simulink model "NREL5MW_Baseline_loads_IPC_1P_v3_2014b"  (R2014b)
settings: Solver=ode3  SolverMode=SingleTasking  StartTime=0.0  StopTime=T-76  RelTol=1e-3
InitFcn:
  | Simsetup
undefined symbols (not defined in the file or in its folder): delta_1p, Demanded_torque, dLP, dLPP, DT, Gainn, IPC_Pitch_max, k_1p, ki_1p, Kp, Mode_gain, NDOF, NumOuts, omega_1p, omega_B, omega_C, omega_L, OutList, PA, Pitch_fine, Pitch_max, Pitch_max_rate, Pitch_min, Pitch_min_rate, PKp, PTi, q_init, qdot_init, strmatch, Ti, Torque_limit, Torque_slew_rate, zeta_1p, zeta_L
libraries: simulink x5
settings Model: ExtModeTrigMode=oneshot  ExtModeArmWhenConnect=off  Creator=Hazim Namik  LastModifiedBy=bwilson
settings OptimizationCC: BlockReduction=off  BooleanDataType=off
settings DebuggingCC: SaveWithParameterizedLinksMsg=none  UnderspecifiedInitializationDetection=Classic  MergeDetectMultiDrivingBlocksExec=none  SignalResolutionControl=TryResolveAllWithWarning  SolverPrmCheckMsg=none  FrameProcessingCompatibilityMsg=error
settings HardwareCC: TargetUnknown=on

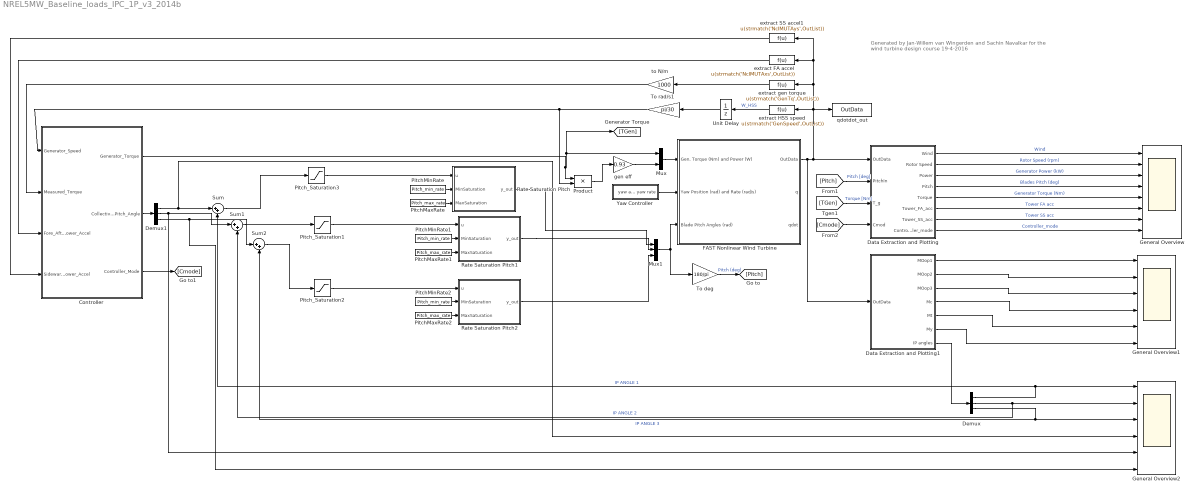
== system NREL5MW_Baseline_loads_IPC_1P_v3_2014b ==
  note: Generated by Jan-Willem van Wingerden and Sachin Navalkar
      | for the wind turbine design course 19-4-2016
  Controller : Subsystem
  Data Extraction and Plotting : Subsystem
  Data Extraction and Plotting1 : Subsystem
  Demux : Demux  Outputs=3
  Demux1 : Demux  Outputs=3
  FAST Nonlinear Wind Turbine : Subsystem  mask(FAST Nonlinear Wind Turbine){}
      mask help: This block contains the FAST S-Function and blocks that integrate the DOF accelerations to get velocities and displacements.
      mask init:
      | clear FAST_SFunc
      settings: MinAlgLoopOccurrences=on
  General Overview : Scope  NumInputPorts=8
      settings: TickLabels=on  YMin=4.47125~10.53034~-754.23394~-1.76549~-5387.5~-3.12398~-0.52601~1.625  YMax=24.47125~15.22691~6788.10547~16.63959~48487.5~2.86069~0.51885~5.375  SaveName=ScopeData2
  General Overview1 : Scope  NumInputPorts=6
      settings: TickLabels=on  YMin=-3775.82161~-2417.73125~-6271.52916~-2978.12919~-4139.15524~-3775.35224  YMax=17382.79924~16229.60392~17181.20499~16116.4566~2206.392~3982.30783
  General Overview2 : Scope  NumInputPorts=6
      settings: TickLabels=on  YMin=-0.04911~-0.0435~-0.0444~-0.02537~-0.02537~-0.02537  YMax=0.04183~0.04676~0.0485~0.24679~0.24679~0.24679
  Mux : Mux  Inputs=2
  Mux1 : Mux  Inputs=3
  PitchMaxRate : Constant  Value=Pitch_max_rate
  PitchMaxRate1 : Constant  Value=Pitch_max_rate
  PitchMaxRate2 : Constant  Value=Pitch_max_rate
  PitchMinRate : Constant  Value=Pitch_min_rate
  PitchMinRate1 : Constant  Value=Pitch_min_rate
  PitchMinRate2 : Constant  Value=Pitch_min_rate
  Pitch_Saturation1 : Saturate  UpperLimit=Pitch_max*pi/180  LowerLimit=Pitch_min*pi/180
  Pitch_Saturation2 : Saturate  UpperLimit=Pitch_max*pi/180  LowerLimit=Pitch_min*pi/180
  Pitch_Saturation3 : Saturate  UpperLimit=Pitch_max*pi/180  LowerLimit=Pitch_min*pi/180
  Product : Product  RndMeth=Zero
  Rate Saturation Pitch : MATLAB Function  TreatAsAtomicUnit=on
  Rate Saturation Pitch1 : MATLAB Function  TreatAsAtomicUnit=on
  Rate Saturation Pitch2 : MATLAB Function  TreatAsAtomicUnit=on
  Sum : Sum  Inputs=|++
  Sum1 : Sum  Inputs=|++
  Sum2 : Sum  Inputs=|++
  To deg : Gain  Gain=180/pi
  To rad/s1 : Gain  Gain=pi/30
  Unit Delay : UnitDelay  InitialCondition=12.1*97  SampleTime=0.0125
  Yaw Controller : Subsystem
  extract FA accel : Fcn  Expr=u(strmatch('NcIMUTAxs',OutList))
  extract HSS speed : Fcn  Expr=u(strmatch('GenSpeed',OutList))
  extract SS accel1 : Fcn  Expr=u(strmatch('NcIMUTAys',OutList))
  extract gen torque : Fcn  Expr=u(strmatch('GenTq',OutList))
  gen eff : Gain  Gain=0.93
  qdotdot_out : ToWorkspace  VariableName=OutData  SampleTime=-1
  to N/m : Gain  Gain=1000
  wires:
  Mux/1 -> FAST Nonlinear Wind Turbine/1(Gen. Torque (Nm) and Power (W))
  Yaw Controller/1(yaw and yaw rate) -> FAST Nonlinear Wind Turbine/2(Yaw Position (rad) and Rate (rad/s))
  extract HSS speed/1 -> Unit Delay/1  "W_HSS"
  To deg/1 -> [Pitch]  "Pitch (deg)"
  gen eff/1 -> Mux/2
  Product/1 -> gen eff/1
  To rad/s1/1 -> Controller/1(Generator_Speed), Product/2
  Data Extraction and Plotting/3(Power) -> General Overview/3  "Generator Power (kW)"
  [Pitch] -> Data Extraction and Plotting/2(PitchIn)  "Pitch [deg]"
  Data Extraction and Plotting/1(Wind) -> General Overview/1  "Wind"
  Data Extraction and Plotting/2(Rotor Speed) -> General Overview/2  "Rotor Speed (rpm)"
  [TGen] -> Data Extraction and Plotting/3(T_g)  "Torque [Nm]"
  FAST Nonlinear Wind Turbine/1(OutData) -> Data Extraction and Plotting1/1(OutData), Data Extraction and Plotting/1(OutData), extract SS accel1/1, extract FA accel/1, extract gen torque/1, extract HSS speed/1, qdotdot_out/1
  Data Extraction and Plotting/4(Pitch) -> General Overview/4  "Blades Pitch (deg)"
  Data Extraction and Plotting/5(Torque) -> General Overview/5  "Generator Torque (Nm)"
  Unit Delay/1 -> To rad/s1/1
  extract gen torque/1 -> to N/m/1
  to N/m/1 -> Controller/2(Measured_Torque)
  Controller/1(Generator_Torque) -> Mux/1, [TGen], Product/1
  extract FA accel/1 -> Controller/3(Fore_Aft_Tower_Accel)
  extract SS accel1/1 -> Controller/4(Sidewards_Tower_Accel)
  Data Extraction and Plotting/6(Tower_FA_acc) -> General Overview/6  "Tower FA acc"
  Data Extraction and Plotting/7(Tower_SS_acc) -> General Overview/7  "Tower SS acc"
  Controller/3(Controller_Mode) -> [Cmode]
  [Cmode] -> Data Extraction and Plotting/4(Cmod)
  Data Extraction and Plotting/8(Controller_mode) -> General Overview/8  "Controller_mode"
  Data Extraction and Plotting1/1(MOop1) -> General Overview1/1
  Data Extraction and Plotting1/2(MOop2) -> General Overview1/2
  Data Extraction and Plotting1/3(MOop3) -> General Overview1/3
  Data Extraction and Plotting1/4(Mc) -> General Overview1/4
  Data Extraction and Plotting1/5(Mt) -> General Overview1/5
  Data Extraction and Plotting1/6(My) -> General Overview1/6
  Data Extraction and Plotting1/7(IP angles) -> Demux/1
  Demux/1 -> Sum/2, General Overview2/1  "IP ANGLE 1"
  Demux/2 -> Sum1/2, General Overview2/2  "IP ANGLE 2"
  Demux/3 -> General Overview2/3, Sum2/2  "IP ANGLE 3"
  Controller/2(Collective_Pitch_Angle) -> Demux1/1
  Demux1/1 -> General Overview2/4, Sum/1
  Demux1/2 -> General Overview2/5, Sum1/1
  Demux1/3 -> General Overview2/6, Sum2/1
  Mux1/1 -> To deg/1, FAST Nonlinear Wind Turbine/3(Blade Pitch Angles (rad))
  Rate Saturation Pitch/1(y_out) -> Mux1/1
  Sum1/1 -> Pitch_Saturation1/1
  Rate Saturation Pitch1/1(y_out) -> Mux1/2
  Rate Saturation Pitch2/1(y_out) -> Mux1/3
  Sum/1 -> Pitch_Saturation3/1
  PitchMinRate/1 -> Rate Saturation Pitch/2(MinSaturation)
  PitchMaxRate/1 -> Rate Saturation Pitch/3(MaxSaturation)
  Pitch_Saturation3/1 -> Rate Saturation Pitch/1(u)
  PitchMinRate1/1 -> Rate Saturation Pitch1/2(MinSaturation)
  PitchMaxRate1/1 -> Rate Saturation Pitch1/3(MaxSaturation)
  Pitch_Saturation1/1 -> Rate Saturation Pitch1/1(u)
  Sum2/1 -> Pitch_Saturation2/1
  PitchMinRate2/1 -> Rate Saturation Pitch2/2(MinSaturation)
  PitchMaxRate2/1 -> Rate Saturation Pitch2/3(MaxSaturation)
  Pitch_Saturation2/1 -> Rate Saturation Pitch2/1(u)

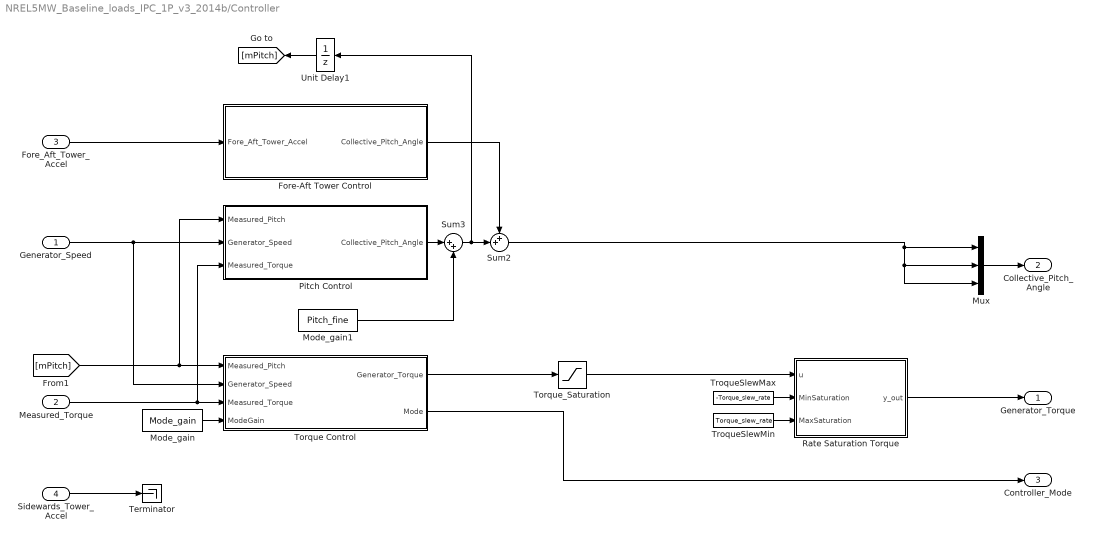
== system NREL5MW_Baseline_loads_IPC_1P_v3_2014b/Controller ==
  Generator_Speed : Inport
  Measured_Torque : Inport  Port=2
  Fore_Aft_Tower_Accel : Inport  Port=3
  Sidewards_Tower_Accel : Inport  Port=4  PortDimensions=1
  Fore-Aft Tower Control : Subsystem
  Mode_gain : Constant  Value=Mode_gain
  Mode_gain1 : Constant  Value=Pitch_fine
  Mux : Mux  Inputs=3
  Pitch Control : Subsystem
  Rate Saturation Torque : MATLAB Function  TreatAsAtomicUnit=on
  Sum2 : Sum  Inputs=++|
  Sum3 : Sum  Inputs=|++
  Terminator : Terminator
  Torque Control : Subsystem
  Torque_Saturation : Saturate  UpperLimit=Torque_limit  LowerLimit=0
  TroqueSlewMax : Constant  Value=-Torque_slew_rate
  TroqueSlewMin : Constant  Value=Torque_slew_rate
  Unit Delay1 : UnitDelay  InitialCondition=12.1*97  SampleTime=DT
  Generator_Torque : Outport
  Collective_Pitch_Angle : Outport  Port=2  PortDimensions=3
  Controller_Mode : Outport  Port=3  PortDimensions=1
  wires:
  Sidewards_Tower_Accel/1 -> Terminator/1
  Fore_Aft_Tower_Accel/1 -> Fore-Aft Tower Control/1(Fore_Aft_Tower_Accel)
  Fore-Aft Tower Control/1(Collective_Pitch_Angle) -> Sum2/1
  Rate Saturation Torque/1(y_out) -> Generator_Torque/1
  [mPitch] -> Pitch Control/1(Measured_Pitch), Torque Control/1(Measured_Pitch)
  Measured_Torque/1 -> Torque Control/3(Measured_Torque), Pitch Control/3(Measured_Torque)
  Generator_Speed/1 -> Pitch Control/2(Generator_Speed), Torque Control/2(Generator_Speed)
  Mode_gain/1 -> Torque Control/4(ModeGain)
  Torque Control/1(Generator_Torque) -> Torque_Saturation/1
  Mux/1 -> Collective_Pitch_Angle/1
  Unit Delay1/1 -> [mPitch]
  Torque Control/2(Mode) -> Controller_Mode/1
  Mode_gain1/1 -> Sum3/2
  Pitch Control/1(Collective_Pitch_Angle) -> Sum3/1
  Sum3/1 -> Sum2/2, Unit Delay1/1
  Sum2/1 -> Mux/2, Mux/3, Mux/1
  Torque_Saturation/1 -> Rate Saturation Torque/1(u)
  TroqueSlewMax/1 -> Rate Saturation Torque/2(MinSaturation)
  TroqueSlewMin/1 -> Rate Saturation Torque/3(MaxSaturation)

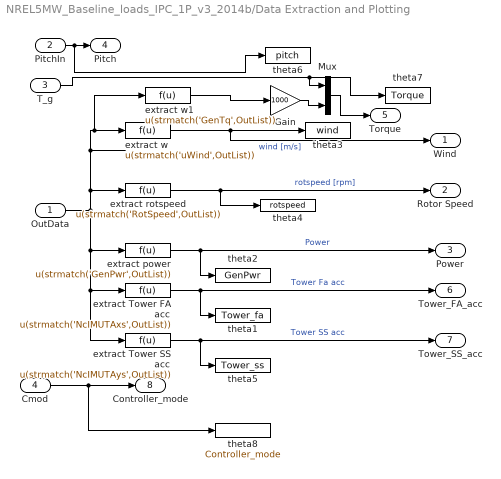
== system NREL5MW_Baseline_loads_IPC_1P_v3_2014b/Data Extraction and Plotting ==
  OutData : Inport
  PitchIn : Inport  Port=2
  T_g : Inport  Port=3
  Cmod : Inport  Port=4
  Gain : Gain  Gain=1000
  Mux : Mux  Inputs=2
  extract Tower FA acc : Fcn  Expr=u(strmatch('NcIMUTAxs',OutList))
  extract Tower SS acc : Fcn  Expr=u(strmatch('NcIMUTAys',OutList))
  extract power : Fcn  Expr=u(strmatch('GenPwr',OutList))
  extract rotspeed : Fcn  Expr=u(strmatch('RotSpeed',OutList))
  extract w : Fcn  Expr=u(strmatch('uWind',OutList))
  extract w1 : Fcn  Expr=u(strmatch('GenTq',OutList))
  theta1 : ToWorkspace  VariableName=Tower_fa
      settings: MaxDataPoints=Inf
  theta2 : ToWorkspace  VariableName=GenPwr
      settings: MaxDataPoints=Inf
  theta3 : ToWorkspace  VariableName=wind
      settings: MaxDataPoints=Inf
  theta4 : ToWorkspace  VariableName=rotspeed
      settings: MaxDataPoints=Inf
  theta5 : ToWorkspace  VariableName=Tower_ss
      settings: MaxDataPoints=Inf
  theta6 : ToWorkspace  VariableName=pitch
      settings: MaxDataPoints=Inf
  theta7 : ToWorkspace  VariableName=Torque
      settings: MaxDataPoints=Inf
  theta8 : ToWorkspace  VariableName=Controller_mode
      settings: MaxDataPoints=Inf
  Wind : Outport
  Rotor Speed : Outport  Port=2
  Power : Outport  Port=3
  Pitch : Outport  Port=4
  Torque : Outport  Port=5
  Tower_FA_acc : Outport  Port=6
  Tower_SS_acc : Outport  Port=7
  Controller_mode : Outport  Port=8
  wires:
  extract w/1 -> Wind/1, theta3/1  "wind [m/s]"
  extract rotspeed/1 -> theta4/1, Rotor Speed/1  "rotspeed [rpm]"
  extract power/1 -> theta2/1, Power/1  "Power"
  PitchIn/1 -> theta6/1, Pitch/1
  T_g/1 -> Mux/1, theta7/1
  extract Tower FA acc/1 -> theta1/1, Tower_FA_acc/1  "Tower Fa acc"
  OutData/1 -> extract w1/1, extract w/1, extract rotspeed/1, extract Tower SS acc/1, extract Tower FA acc/1, extract power/1
  extract Tower SS acc/1 -> theta5/1, Tower_SS_acc/1  "Tower SS acc"
  Cmod/1 -> theta8/1, Controller_mode/1
  extract w1/1 -> Gain/1
  Gain/1 -> Mux/2
  Mux/1 -> Torque/1

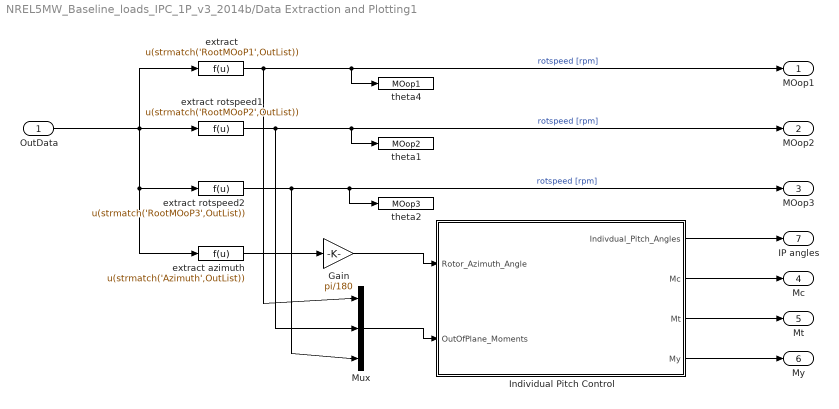
== system NREL5MW_Baseline_loads_IPC_1P_v3_2014b/Data Extraction and Plotting1 ==
  OutData : Inport
  Gain : Gain  Gain=pi/180
  Individual Pitch Control : Subsystem
  Mux : Mux  Inputs=3
  "extract " : Fcn  Expr=u(strmatch('RootMOoP1',OutList))
  extract azimuth : Fcn  Expr=u(strmatch('Azimuth',OutList))
  extract rotspeed1 : Fcn  Expr=u(strmatch('RootMOoP2',OutList))
  extract rotspeed2 : Fcn  Expr=u(strmatch('RootMOoP3',OutList))
  theta1 : ToWorkspace  VariableName=MOop2
      settings: MaxDataPoints=Inf
  theta2 : ToWorkspace  VariableName=MOop3
      settings: MaxDataPoints=Inf
  theta4 : ToWorkspace  VariableName=MOop1
      settings: MaxDataPoints=Inf
  MOop1 : Outport
  MOop2 : Outport  Port=2
  MOop3 : Outport  Port=3
  Mc : Outport  Port=4
  Mt : Outport  Port=5
  My : Outport  Port=6
  IP angles : Outport  Port=7
  wires:
  "extract "/1 -> Mux/1, theta4/1, MOop1/1  "rotspeed [rpm]"
  extract rotspeed1/1 -> Mux/2, theta1/1, MOop2/1  "rotspeed [rpm]"
  extract rotspeed2/1 -> theta2/1, MOop3/1, Mux/3  "rotspeed [rpm]"
  OutData/1 -> "extract "/1, extract azimuth/1, extract rotspeed2/1, extract rotspeed1/1
  Mux/1 -> Individual Pitch Control/2(OutOfPlane_Moments)
  extract azimuth/1 -> Gain/1
  Individual Pitch Control/2(Mc) -> Mc/1
  Individual Pitch Control/3(Mt) -> Mt/1
  Individual Pitch Control/4(My) -> My/1
  Gain/1 -> Individual Pitch Control/1(Rotor_Azimuth_Angle)
  Individual Pitch Control/1(Indivdual_Pitch_Angles) -> IP angles/1

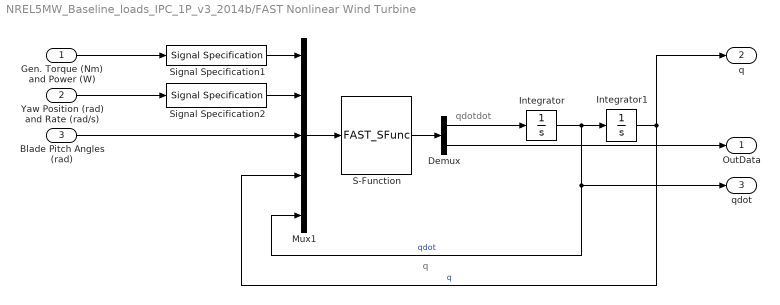
== system NREL5MW_Baseline_loads_IPC_1P_v3_2014b/FAST Nonlinear Wind Turbine ==
  note: qdotdot
  note: q
  Gen. Torque (Nm) and Power (W) : Inport
  Yaw Position (rad) and Rate (rad/s) : Inport  Port=2
  Blade Pitch Angles (rad) : Inport  Port=3
  Demux : Demux  Outputs=[NDOF, NumOuts]
  Integrator : Integrator  InitialCondition=qdot_init
  Integrator1 : Integrator  InitialCondition=q_init
  Mux1 : Mux  Inputs=5
  S-Function : S-Function  FunctionName=FAST_SFunc  EnableBusSupport=off
  Signal Specification1 : SignalSpecification  OutDataTypeStr=double  Dimensions=2
  Signal Specification2 : SignalSpecification  OutDataTypeStr=double  Dimensions=2
  OutData : Outport
  q : Outport  Port=2
  qdot : Outport  Port=3
  wires:
  Integrator/1 -> Integrator1/1, Mux1/5, qdot/1  "qdot"
  Gen. Torque (Nm) and Power (W)/1 -> Signal Specification1/1
  S-Function/1 -> Demux/1
  Demux/1 -> Integrator/1
  Demux/2 -> OutData/1
  Mux1/1 -> S-Function/1
  Blade Pitch Angles (rad)/1 -> Mux1/3
  Yaw Position (rad) and Rate (rad/s)/1 -> Signal Specification2/1
  Integrator1/1 -> Mux1/4, q/1  "q"
  Signal Specification1/1 -> Mux1/1
  Signal Specification2/1 -> Mux1/2

== system NREL5MW_Baseline_loads_IPC_1P_v3_2014b/Yaw Controller ==
  Mux : Mux  Inputs=2
  Yaw Position : Constant  Value=0
  Yaw rate : Constant  Value=0
  yaw and yaw rate : Outport
  wires:
  Mux/1 -> yaw and yaw rate/1
  Yaw Position/1 -> Mux/1
  Yaw rate/1 -> Mux/2

== system NREL5MW_Baseline_loads_IPC_1P_v3_2014b/Controller/Fore-Aft Tower Control ==
  note: Fore-Aft tower damping
  Fore_Aft_Tower_Accel : Inport
  Discrete-Time Integrator : DiscreteIntegrator  SampleTime=DT
  Gain : Gain  Gain=Gainn
  Pitch_Saturation : Saturate  UpperLimit=Pitch_max*pi/180  LowerLimit=Pitch_min*pi/180
  Collective_Pitch_Angle : Outport
  wires:
  Fore_Aft_Tower_Accel/1 -> Discrete-Time Integrator/1
  Pitch_Saturation/1 -> Collective_Pitch_Angle/1
  Discrete-Time Integrator/1 -> Gain/1
  Gain/1 -> Pitch_Saturation/1

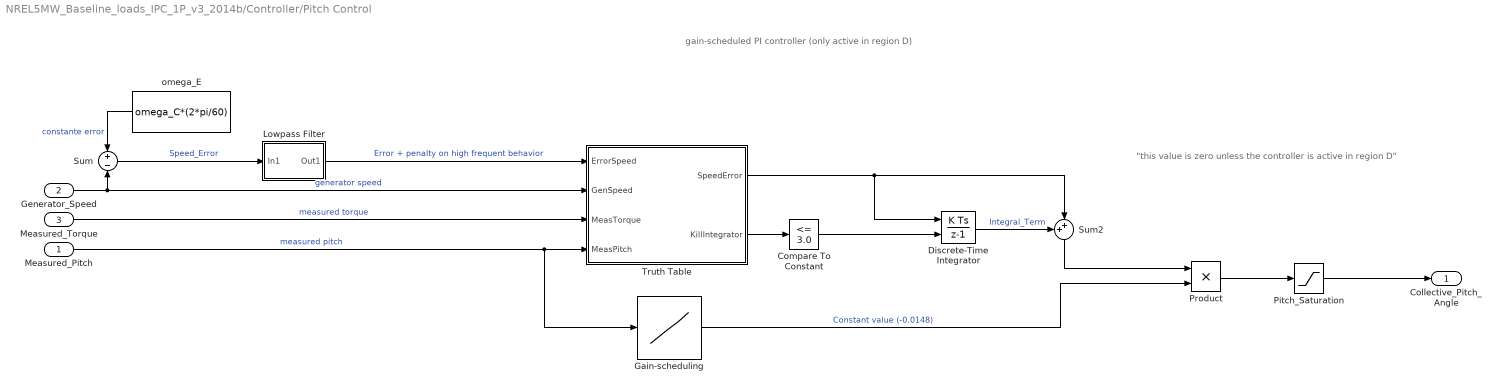
== system NREL5MW_Baseline_loads_IPC_1P_v3_2014b/Controller/Pitch Control ==
  note: gain-scheduled PI controller (only active in region D)
  note: "this value is zero unless the controller is active in region D"
  Measured_Pitch : Inport
  Generator_Speed : Inport  Port=2
  Measured_Torque : Inport  Port=3
  Compare To Constant : simulink/Logic and Bit Operations/Compare To Constant  relop=<=  const=3.0  OutDataTypeStr=boolean
  Discrete-Time Integrator : DiscreteIntegrator  gainval=PTi(1)  ExternalReset=level  InitialConditionSetting=State (most efficient)  SampleTime=DT
  Gain-scheduling : Lookup  InputValues=PA  Table=PKp
  Lowpass Filter : Subsystem
  Pitch_Saturation : Saturate  UpperLimit=Pitch_max*pi/180  LowerLimit=Pitch_min*pi/180
  Product : Product  RndMeth=Zero
  Sum : Sum  Inputs=+-
  Sum2 : Sum  Inputs=++|
  Truth Table : Truth Table  TreatAsAtomicUnit=on
  omega_E : Constant  Value=omega_C*(2*pi/60)
  Collective_Pitch_Angle : Outport
  wires:
  Discrete-Time Integrator/1 -> Sum2/1  "Integral_Term"
  Sum2/1 -> Product/1
  Measured_Pitch/1 -> Gain-scheduling/1, Truth Table/4(MeasPitch)  "measured pitch"
  Gain-scheduling/1 -> Product/2  "Constant value (-0.0148)"
  Generator_Speed/1 -> Truth Table/2(GenSpeed), Sum/2  "generator speed"
  Truth Table/1(SpeedError) -> Sum2/2, Discrete-Time Integrator/1
  Measured_Torque/1 -> Truth Table/3(MeasTorque)  "measured torque"
  Pitch_Saturation/1 -> Collective_Pitch_Angle/1
  Compare To Constant/1 -> Discrete-Time Integrator/2
  Truth Table/2(KillIntegrator) -> Compare To Constant/1
  Product/1 -> Pitch_Saturation/1
  Sum/1 -> Lowpass Filter/1(In1)  "Speed_Error"
  Lowpass Filter/1(Out1) -> Truth Table/1(ErrorSpeed)  "Error + penalty on high frequent behavior"
  omega_E/1 -> Sum/1  "constante error"

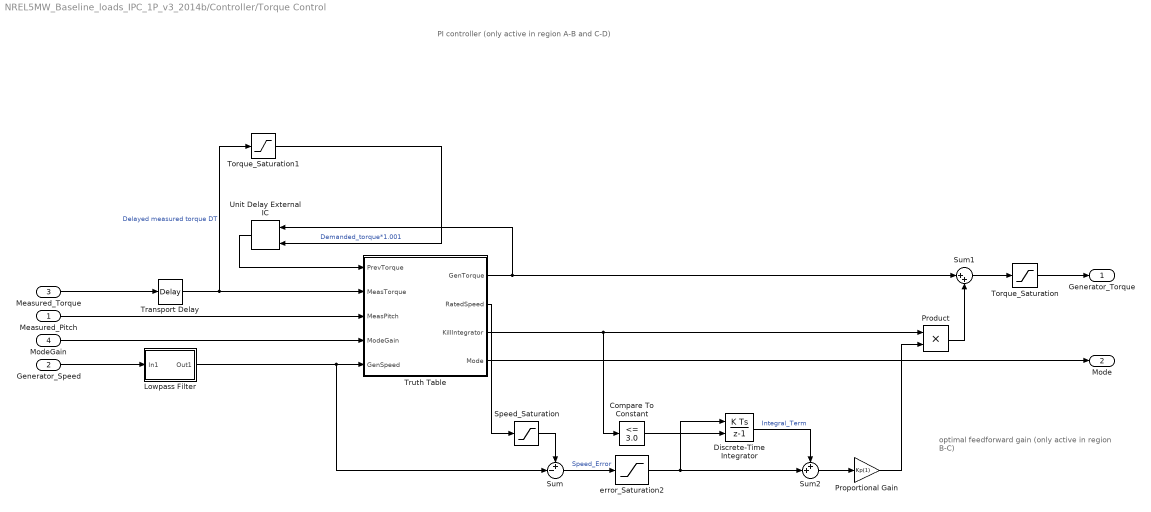
== system NREL5MW_Baseline_loads_IPC_1P_v3_2014b/Controller/Torque Control ==
  note: PI controller
      | (only active in region A-B and C-D)
  note: optimal feedforward gain
      | (only active in region B-C)
  Measured_Pitch : Inport
  Generator_Speed : Inport  Port=2
  Measured_Torque : Inport  Port=3
  ModeGain : Inport  Port=4
  Compare To Constant : simulink/Logic and Bit Operations/Compare To Constant  relop=<=  const=3.0  OutDataTypeStr=boolean
  Discrete-Time Integrator : DiscreteIntegrator  gainval=Ti(1)  ExternalReset=level  SampleTime=DT  UpperSaturationLimit=12000/2300  LowerSaturationLimit=-12000/2300
  Lowpass Filter : Subsystem
  Product : Product  RndMeth=Zero
  Proportional Gain : Gain  Gain=Kp(1)
  Speed_Saturation : Saturate  UpperLimit=omega_C*(2*pi/60)  LowerLimit=-100
  Sum : Sum  Inputs=+-|
  Sum1 : Sum  Inputs=|++
  Sum2 : Sum  Inputs=++|
  Torque_Saturation : Saturate  UpperLimit=Torque_limit*1.001  LowerLimit=0
  Torque_Saturation1 : Saturate  UpperLimit=Demanded_torque*1.001;  LowerLimit=0
  Transport Delay : TransportDelay  DelayTime=DT
  Truth Table : Truth Table  TreatAsAtomicUnit=on
  Unit Delay External IC : simulink/Additional Math & Discrete/Additional Discrete/Unit Delay External IC  tsamp=-1
  error_Saturation2 : Saturate  UpperLimit=0  LowerLimit=-1e14
  Generator_Torque : Outport
  Mode : Outport  Port=2
  wires:
  Measured_Torque/1 -> Transport Delay/1
  Sum2/1 -> Proportional Gain/1
  Generator_Speed/1 -> Lowpass Filter/1(In1)
  Truth Table/2(RatedSpeed) -> Speed_Saturation/1
  Truth Table/1(GenTorque) -> Unit Delay External IC/1, Sum1/1
  Torque_Saturation/1 -> Generator_Torque/1
  Sum1/1 -> Torque_Saturation/1
  Truth Table/3(KillIntegrator) -> Compare To Constant/1, Product/1
  Discrete-Time Integrator/1 -> Sum2/1  "Integral_Term"
  Product/1 -> Sum1/2
  Proportional Gain/1 -> Product/2
  Compare To Constant/1 -> Discrete-Time Integrator/2
  Unit Delay External IC/1 -> Truth Table/1(PrevTorque)
  Lowpass Filter/1(Out1) -> Sum/2, Truth Table/5(GenSpeed)
  Speed_Saturation/1 -> Sum/1
  Torque_Saturation1/1 -> Unit Delay External IC/2  "Demanded_torque*1.001"
  Sum/1 -> error_Saturation2/1  "Speed_Error"
  error_Saturation2/1 -> Sum2/2, Discrete-Time Integrator/1
  Truth Table/4(Mode) -> Mode/1
  Measured_Pitch/1 -> Truth Table/3(MeasPitch)
  Transport Delay/1 -> Truth Table/2(MeasTorque), Torque_Saturation1/1  "Delayed measured torque DT"
  ModeGain/1 -> Truth Table/4(ModeGain)

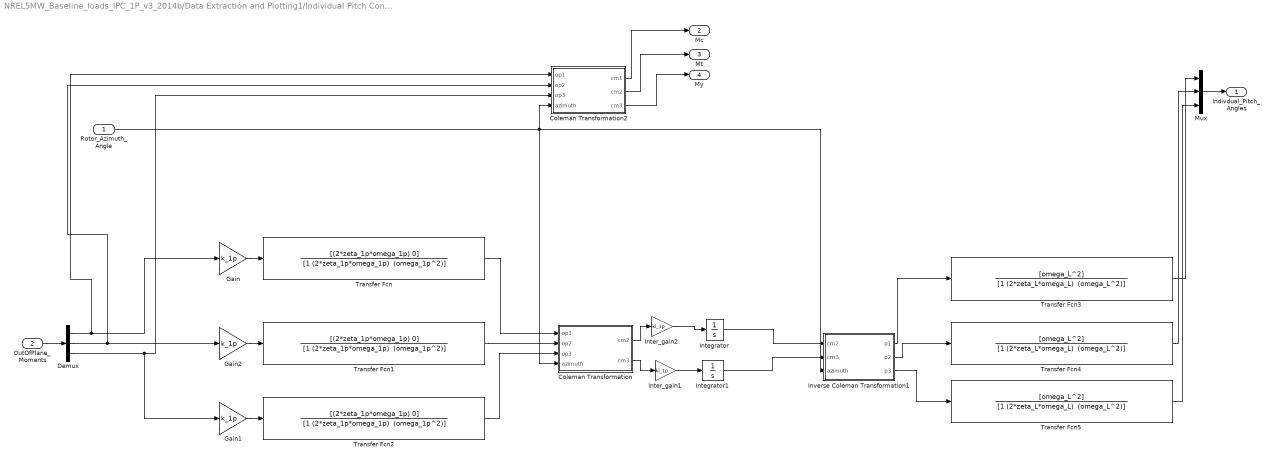
== system NREL5MW_Baseline_loads_IPC_1P_v3_2014b/Data Extraction and Plotting1/Individual Pitch Control ==
  Rotor_Azimuth_Angle : Inport
  OutOfPlane_Moments : Inport  Port=2
  Coleman Transformation : Subsystem
  Coleman Transformation2 : Subsystem
  Demux : Demux  Outputs=3
  Gain : Gain  Gain=k_1p
  Gain1 : Gain  Gain=k_1p
  Gain2 : Gain  Gain=k_1p
  Integrator : Integrator  LimitOutput=on  UpperSaturationLimit=IPC_Pitch_max*pi/180  LowerSaturationLimit=-IPC_Pitch_max*pi/180
  Integrator1 : Integrator  LimitOutput=on  UpperSaturationLimit=IPC_Pitch_max*pi/180  LowerSaturationLimit=-IPC_Pitch_max*pi/180
  Inter_gain1 : Gain  Gain=ki_1p
  Inter_gain2 : Gain  Gain=ki_1p
  Inverse Coleman Transformation1 : Subsystem
  Mux : Mux  Inputs=3
  Transfer Fcn : TransferFcn  Numerator=[(2*zeta_1p*omega_1p) 0]  Denominator="[1 (2*zeta_1p*omega_1p)  (omega_1p^2)]"
  Transfer Fcn1 : TransferFcn  Numerator=[(2*zeta_1p*omega_1p) 0]  Denominator="[1 (2*zeta_1p*omega_1p)  (omega_1p^2)]"
  Transfer Fcn2 : TransferFcn  Numerator=[(2*zeta_1p*omega_1p) 0]  Denominator="[1 (2*zeta_1p*omega_1p)  (omega_1p^2)]"
  Transfer Fcn3 : TransferFcn  Numerator=[omega_L^2]  Denominator="[1 (2*zeta_L*omega_L)  (omega_L^2)]"
  Transfer Fcn4 : TransferFcn  Numerator=[omega_L^2]  Denominator="[1 (2*zeta_L*omega_L)  (omega_L^2)]"
  Transfer Fcn5 : TransferFcn  Numerator=[omega_L^2]  Denominator="[1 (2*zeta_L*omega_L)  (omega_L^2)]"
  Indivdual_Pitch_Angles : Outport
  Mc : Outport  Port=2
  Mt : Outport  Port=3
  My : Outport  Port=4
  wires:
  Mux/1 -> Indivdual_Pitch_Angles/1
  OutOfPlane_Moments/1 -> Demux/1
  Rotor_Azimuth_Angle/1 -> Inverse Coleman Transformation1/3(azimuth), Coleman Transformation2/4(azimuth), Coleman Transformation/4(azimuth)
  Coleman Transformation/1(cm2) -> Inter_gain2/1
  Inter_gain2/1 -> Integrator/1
  Coleman Transformation/2(cm3) -> Inter_gain1/1
  Inter_gain1/1 -> Integrator1/1
  Gain/1 -> Transfer Fcn/1
  Demux/1 -> Coleman Transformation2/1(op1), Gain/1
  Transfer Fcn/1 -> Coleman Transformation/1(op1)
  Gain1/1 -> Transfer Fcn2/1
  Demux/3 -> Coleman Transformation2/3(op3), Gain1/1
  Transfer Fcn2/1 -> Coleman Transformation/3(op3)
  Gain2/1 -> Transfer Fcn1/1
  Demux/2 -> Coleman Transformation2/2(op2), Gain2/1
  Transfer Fcn1/1 -> Coleman Transformation/2(op2)
  Inverse Coleman Transformation1/1(p1) -> Transfer Fcn3/1
  Inverse Coleman Transformation1/2(p2) -> Transfer Fcn4/1
  Inverse Coleman Transformation1/3(p3) -> Transfer Fcn5/1
  Coleman Transformation2/1(cm1) -> Mc/1
  Coleman Transformation2/2(cm2) -> Mt/1
  Coleman Transformation2/3(cm3) -> My/1
  Transfer Fcn3/1 -> Mux/1
  Transfer Fcn4/1 -> Mux/2
  Transfer Fcn5/1 -> Mux/3
  Integrator/1 -> Inverse Coleman Transformation1/1(cm2)
  Integrator1/1 -> Inverse Coleman Transformation1/2(cm3)

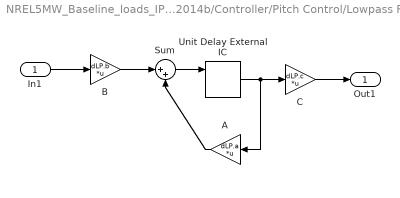
== system NREL5MW_Baseline_loads_IPC_1P_v3_2014b/Controller/Pitch Control/Lowpass Filter ==
  In1 : Inport
  A : Gain  Gain=dLP.a  Multiplication=Matrix(K*u) (u vector)
  B : Gain  Gain=dLP.b  Multiplication=Matrix(K*u) (u vector)
  C : Gain  Gain=dLP.c  Multiplication=Matrix(K*u) (u vector)
  Sum : Sum  Inputs=|++
  Unit Delay External IC : simulink/Additional Math & Discrete/Additional Discrete/Unit Delay External IC  tsamp=-1
  Out1 : Outport
  wires:
  In1/1 -> B/1
  C/1 -> Out1/1
  Unit Delay External IC/1 -> C/1, A/1
  B/1 -> Sum/1
  Sum/1 -> Unit Delay External IC/1
  A/1 -> Sum/2

== system NREL5MW_Baseline_loads_IPC_1P_v3_2014b/Controller/Torque Control/Lowpass Filter ==
  In1 : Inport
  A : Gain  Gain=dLPP.a  Multiplication=Matrix(K*u)
  B : Gain  Gain=dLPP.b  Multiplication=Matrix(K*u)
  C : Gain  Gain=dLPP.c  Multiplication=Matrix(K*u)
  Sum : Sum  Inputs=|++
  Unit Delay External IC : simulink/Additional Math & Discrete/Additional Discrete/Unit Delay External IC  tsamp=-1
  Out1 : Outport
  wires:
  In1/1 -> B/1
  C/1 -> Out1/1
  Unit Delay External IC/1 -> C/1, A/1
  B/1 -> Sum/1
  Sum/1 -> Unit Delay External IC/1
  A/1 -> Sum/2

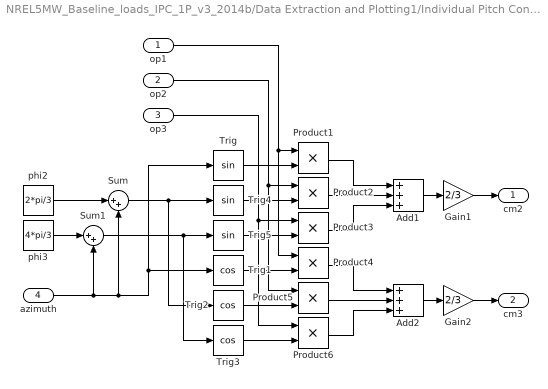
== system NREL5MW_Baseline_loads_IPC_1P_v3_2014b/Data Extraction and Plotting1/Individual Pitch Control/Coleman Transformation ==
  op1 : Inport
  op2 : Inport  Port=2
  op3 : Inport  Port=3
  azimuth : Inport  Port=4
  Add1 : Sum  Inputs=+++
  Add2 : Sum  Inputs=+++
  Gain1 : Gain  Gain=2/3
  Gain2 : Gain  Gain=2/3
  Product{1..6} (6 alike) : Product  RndMeth=Zero
  Sum : Sum  Inputs=|++
  Sum1 : Sum  Inputs=|++
  Trig : Trigonometry
  Trig1 : Trigonometry  Operator=cos
  Trig2 : Trigonometry  Operator=cos
  Trig3 : Trigonometry  Operator=cos
  Trig4 : Trigonometry
  Trig5 : Trigonometry
  phi2 : Constant  Value=2*pi/3
  phi3 : Constant  Value=4*pi/3
  cm2 : Outport
  cm3 : Outport  Port=2
  wires:
  Add1/1 -> Gain1/1
  phi2/1 -> Sum/1
  phi3/1 -> Sum1/1
  azimuth/1 -> Sum1/2, Sum/2, Trig/1, Trig1/1
  Trig/1 -> Product1/2
  Trig4/1 -> Product2/2
  Trig5/1 -> Product3/2
  Trig1/1 -> Product4/2
  Trig2/1 -> Product5/2
  Trig3/1 -> Product6/2
  Sum/1 -> Trig4/1, Trig2/1
  Sum1/1 -> Trig5/1, Trig3/1
  Add2/1 -> Gain2/1
  Gain1/1 -> cm2/1
  Gain2/1 -> cm3/1
  op1/1 -> Product1/1, Product4/1
  op2/1 -> Product2/1, Product5/1
  op3/1 -> Product6/1, Product3/1
  Product1/1 -> Add1/1
  Product2/1 -> Add1/2
  Product3/1 -> Add1/3
  Product4/1 -> Add2/1
  Product5/1 -> Add2/2
  Product6/1 -> Add2/3

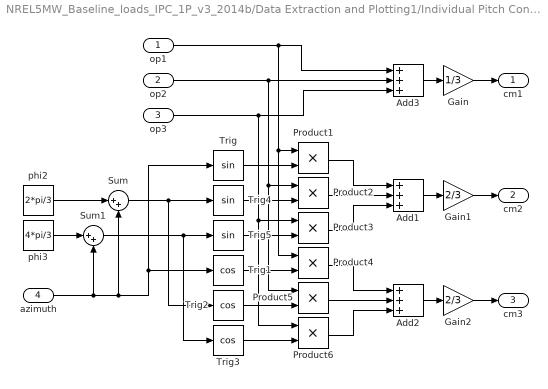
== system NREL5MW_Baseline_loads_IPC_1P_v3_2014b/Data Extraction and Plotting1/Individual Pitch Control/Coleman Transformation2 ==
  op1 : Inport
  op2 : Inport  Port=2
  op3 : Inport  Port=3
  azimuth : Inport  Port=4
  Add1 : Sum  Inputs=+++
  Add2 : Sum  Inputs=+++
  Add3 : Sum  Inputs=+++
  Gain : Gain  Gain=1/3
  Gain1 : Gain  Gain=2/3
  Gain2 : Gain  Gain=2/3
  Product{1..6} (6 alike) : Product  RndMeth=Zero
  Sum : Sum  Inputs=|++
  Sum1 : Sum  Inputs=|++
  Trig : Trigonometry
  Trig1 : Trigonometry  Operator=cos
  Trig2 : Trigonometry  Operator=cos
  Trig3 : Trigonometry  Operator=cos
  Trig4 : Trigonometry
  Trig5 : Trigonometry
  phi2 : Constant  Value=2*pi/3
  phi3 : Constant  Value=4*pi/3
  cm1 : Outport
  cm2 : Outport  Port=2
  cm3 : Outport  Port=3
  wires:
  Add1/1 -> Gain1/1
  phi2/1 -> Sum/1
  phi3/1 -> Sum1/1
  azimuth/1 -> Sum1/2, Sum/2, Trig/1, Trig1/1
  Trig/1 -> Product1/2
  Trig4/1 -> Product2/2
  Trig5/1 -> Product3/2
  Trig1/1 -> Product4/2
  Trig2/1 -> Product5/2
  Trig3/1 -> Product6/2
  Sum/1 -> Trig4/1, Trig2/1
  Sum1/1 -> Trig5/1, Trig3/1
  Add2/1 -> Gain2/1
  Add3/1 -> Gain/1
  Gain/1 -> cm1/1
  Gain1/1 -> cm2/1
  Gain2/1 -> cm3/1
  op1/1 -> Add3/1, Product1/1, Product4/1
  op2/1 -> Add3/2, Product2/1, Product5/1
  op3/1 -> Add3/3, Product6/1, Product3/1
  Product1/1 -> Add1/1
  Product2/1 -> Add1/2
  Product3/1 -> Add1/3
  Product4/1 -> Add2/1
  Product5/1 -> Add2/2
  Product6/1 -> Add2/3

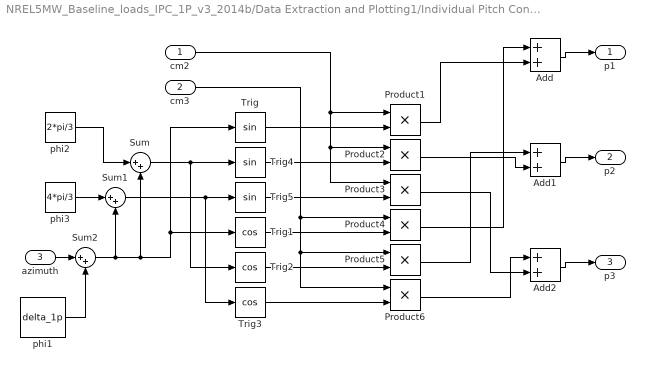
== system NREL5MW_Baseline_loads_IPC_1P_v3_2014b/Data Extraction and Plotting1/Individual Pitch Control/Inverse Coleman Transformation1 ==
  cm2 : Inport
  cm3 : Inport  Port=2
  azimuth : Inport  Port=3
  Add : Sum
  Add1 : Sum
  Add2 : Sum
  Product{1..6} (6 alike) : Product  RndMeth=Zero
  Sum : Sum  Inputs=|++
  Sum1 : Sum  Inputs=|++
  Sum2 : Sum  Inputs=|++
  Trig : Trigonometry
  Trig1 : Trigonometry  Operator=cos
  Trig2 : Trigonometry  Operator=cos
  Trig3 : Trigonometry  Operator=cos
  Trig4 : Trigonometry
  Trig5 : Trigonometry
  phi1 : Constant  Value=delta_1p
  phi2 : Constant  Value=2*pi/3
  phi3 : Constant  Value=4*pi/3
  p1 : Outport
  p2 : Outport  Port=2
  p3 : Outport  Port=3
  wires:
  phi2/1 -> Sum/1
  phi3/1 -> Sum1/1
  Sum2/1 -> Sum1/2, Sum/2, Trig/1, Trig1/1
  Sum/1 -> Trig4/1, Trig2/1
  Sum1/1 -> Trig5/1, Trig3/1
  Add/1 -> p1/1
  Add1/1 -> p2/1
  Add2/1 -> p3/1
  Trig/1 -> Product1/2
  Trig4/1 -> Product2/2
  Trig5/1 -> Product3/2
  Trig1/1 -> Product4/2
  Trig2/1 -> Product5/2
  Trig3/1 -> Product6/2
  cm2/1 -> Product1/1, Product2/1, Product3/1
  Product1/1 -> Add/2
  Product2/1 -> Add1/2
  Product3/1 -> Add2/2
  cm3/1 -> Product4/1, Product5/1, Product6/1
  Product4/1 -> Add/1
  Product5/1 -> Add1/1
  Product6/1 -> Add2/1
  phi1/1 -> Sum2/2
  azimuth/1 -> Sum2/1

== matlab function NREL5MW_Baseline_loads_IPC_1P_v3_2014b/Controller/Rate Saturation Torque ==
  data: u input; MinSaturation input; y_out output; MaxSaturation input; DT parameter
function y_out = fcn(u,MinSaturation,MaxSaturation,DT)
persistent y

if isempty(y)
    y = u;
end

rate = (u-y)/DT;
rate = min(max(rate,MinSaturation),MaxSaturation);

y = y + rate*DT;
y_out = y;

== matlab function NREL5MW_Baseline_loads_IPC_1P_v3_2014b/Rate Saturation Pitch ==
  data: u input; MinSaturation input; y_out output; MaxSaturation input; DT parameter
function y_out = fcn(u,MinSaturation,MaxSaturation,DT)
persistent y

if isempty(y)
    y = u;
end

rate = (u-y)/DT;
rate = min(max(rate,MinSaturation),MaxSaturation);

y = y + rate*DT;
y_out = y;

== matlab function NREL5MW_Baseline_loads_IPC_1P_v3_2014b/Controller/Pitch Control/Truth Table ==
  data: ErrorSpeed input; SpeedError output; GenSpeed input double; MeasTorque input double; MeasPitch input double; KillIntegrator output double; omega_C local double; Demanded_torque parameter double
function [SpeedError, KillIntegrator] = fcn(ErrorSpeed, GenSpeed, MeasTorque, MeasPitch, Demanded_torque)

aVarTruthTableCondition_1 = false;
aVarTruthTableCondition_2 = false;


% Measured Speed

aVarTruthTableCondition_1 = logical(GenSpeed >= omega_C*(2*pi/60));

% Measured torque

aVarTruthTableCondition_2 = logical(MeasTorque >= Demanded_torque*0.999);

if (~aVarTruthTableCondition_1 && ~aVarTruthTableCondition_2)
    aFcnTruthTableAction_1();
elseif (~aVarTruthTableCondition_1 && aVarTruthTableCondition_2)
    aFcnTruthTableAction_1();
elseif (aVarTruthTableCondition_1 && ~aVarTruthTableCondition_2)
    aFcnTruthTableAction_1();
else % Default
    aFcnTruthTableAction_2();
end

function aFcnTruthTableAction_1()

% No Pitching

SpeedError = 0;
KillIntegrator = 0;

function aFcnTruthTableAction_2()

% Pitching

SpeedError = ErrorSpeed;
KillIntegrator = 1;

== matlab function NREL5MW_Baseline_loads_IPC_1P_v3_2014b/Controller/Torque Control/Truth Table ==
  data: PrevTorque input double; MeasTorque input double; MeasPitch input double; ModeGain input double; GenSpeed input; GenTorque output; RatedSpeed output double; KillIntegrator output double; omega_A constant double; omega_B parameter double; omega_C parameter double; Demanded_torque parameter double; Mode output double; Pitch_fine parameter double
function [GenTorque, RatedSpeed, KillIntegrator, Mode] = fcn(PrevTorque, MeasTorque, MeasPitch, ModeGain, GenSpeed, omega_B, omega_C, Demanded_torque, Pitch_fine)

aVarTruthTableCondition_1 = false;
aVarTruthTableCondition_2 = false;
aVarTruthTableCondition_3 = false;
aVarTruthTableCondition_4 = false;
aVarTruthTableCondition_5 = false;
aVarTruthTableCondition_6 = false;
aVarTruthTableCondition_7 = false;


% No operation

aVarTruthTableCondition_1 = logical(GenSpeed < omega_A*(2*pi/60));

% Region A-B

aVarTruthTableCondition_2 = logical(GenSpeed < omega_B*(2*pi/60));

% Region A-B

aVarTruthTableCondition_3 = logical(MeasTorque < ModeGain*omega_B*(2*pi/60)*omega_B*(2*pi/60));

% Region B-C

aVarTruthTableCondition_4 = logical(GenSpeed < omega_C*(2*pi/60));

% Region B-C

aVarTruthTableCondition_5 = logical(MeasTorque < ModeGain*omega_C*(2*pi/60)*omega_C*(2*pi/60));

% Region C-D

aVarTruthTableCondition_6 = logical(MeasTorque < Demanded_torque);

% Pitch Command

aVarTruthTableCondition_7 = logical(MeasPitch > Pitch_fine*1.05);

if (aVarTruthTableCondition_1)
    aFcnTruthTableAction_1();
elseif (~aVarTruthTableCondition_1 && aVarTruthTableCondition_2 && aVarTruthTableCondition_3)
    aFcnTruthTableAction_2();
elseif (~aVarTruthTableCondition_1 && aVarTruthTableCondition_2 && ~aVarTruthTableCondition_3)
    aFcnTruthTableAction_2();
elseif (~aVarTruthTableCondition_1 && ~aVarTruthTableCondition_2 && aVarTruthTableCondition_3 && aVarTruthTableCondition_4)
    aFcnTruthTableAction_2();
elseif (~aVarTruthTableCondition_1 && ~aVarTruthTableCondition_2 && aVarTruthTableCondition_3 && ~aVarTruthTableCondition_4)
    aFcnTruthTableAction_3();
elseif (~aVarTruthTableCondition_1 && ~aVarTruthTableCondition_2 && ~aVarTruthTableCondition_3 && aVarTruthTableCondition_4 && aVarTruthTableCondition_5)
    aFcnTruthTableAction_3();
elseif (~aVarTruthTableCondition_1 && ~aVarTruthTableCondition_2 && ~aVarTruthTableCondition_3 && ~aVarTruthTableCondition_4 && aVarTruthTableCondition_5)
    aFcnTruthTableAction_4();
elseif (~aVarTruthTableCondition_1 && ~aVarTruthTableCondition_2 && ~aVarTruthTableCondition_3 && aVarTruthTableCondition_4 && ~aVarTruthTableCondition_5 && aVarTruthTableCondition_6 && aVarTruthTableCondition_7)
    aFcnTruthTableAction_4();
elseif (~aVarTruthTableCondition_1 && ~aVarTruthTableCondition_2 && ~aVarTruthTableCondition_3 && aVarTruthTableCondition_4 && ~aVarTruthTableCondition_5 && aVarTruthTableCondition_6 && ~aVarTruthTableCondition_7)
    aFcnTruthTableAction_4();
elseif (~aVarTruthTableCondition_1 && ~aVarTruthTableCondition_2 && ~aVarTruthTableCondition_3 && aVarTruthTableCondition_4 && ~aVarTruthTableCondition_5 && ~aVarTruthTableCondition_6 && aVarTruthTableCondition_7)
    aFcnTruthTableAction_5();
elseif (~aVarTruthTableCondition_1 && ~aVarTruthTableCondition_2 && ~aVarTruthTableCondition_3 && aVarTruthTableCondition_4 && ~aVarTruthTableCondition_5 && ~aVarTruthTableCondition_6 && ~aVarTruthTableCondition_7)
    aFcnTruthTableAction_4();
elseif (~aVarTruthTableCondition_1 && ~aVarTruthTableCondition_2 && ~aVarTruthTableCondition_3 && ~aVarTruthTableCondition_4 && ~aVarTruthTableCondition_5 && aVarTruthTableCondition_6 && aVarTruthTableCondition_7)
    aFcnTruthTableAction_5();
elseif (~aVarTruthTableCondition_1 && ~aVarTruthTableCondition_2 && ~aVarTruthTableCondition_3 && ~aVarTruthTableCondition_4 && ~aVarTruthTableCondition_5 && aVarTruthTableCondition_6 && ~aVarTruthTableCondition_7)
    aFcnTruthTableAction_4();
elseif (~aVarTruthTableCondition_1 && ~aVarTruthTableCondition_2 && ~aVarTruthTableCondition_3 && ~aVarTruthTableCondition_4 && ~aVarTruthTableCondition_5 && ~aVarTruthTableCondition_6 && aVarTruthTableCondition_7)
    aFcnTruthTableAction_5();
else % Default
    aFcnTruthTableAction_5();
end

function aFcnTruthTableAction_1()

% No operation

RatedSpeed = GenSpeed;
GenTorque = 0;
KillIntegrator = 0;
Mode=1;

function aFcnTruthTableAction_2()

% Region A-B

RatedSpeed = omega_B*(2*pi/60);
GenTorque = PrevTorque;
KillIntegrator = 1;
Mode=2;

function aFcnTruthTableAction_3()

% Region B-C

RatedSpeed = GenSpeed;
GenTorque = ModeGain*GenSpeed*GenSpeed;
KillIntegrator = 0;
Mode=3;

function aFcnTruthTableAction_4()

% Region C-D

RatedSpeed = omega_C*(2*pi/60);
GenTorque = PrevTorque;
KillIntegrator = 1;
Mode=4;

function aFcnTruthTableAction_5()

% Region D

RatedSpeed = GenSpeed;
GenTorque = Demanded_torque;
KillIntegrator = 0;
Mode=5;

== matlab function NREL5MW_Baseline_loads_IPC_1P_v3_2014b/Rate Saturation Pitch1 ==
  data: u input; MinSaturation input; y_out output; MaxSaturation input; DT parameter
function y_out = fcn(u,MinSaturation,MaxSaturation,DT)
persistent y

if isempty(y)
    y = u;
end

rate = (u-y)/DT;
rate = min(max(rate,MinSaturation),MaxSaturation);

y = y + rate*DT;
y_out = y;

== matlab function NREL5MW_Baseline_loads_IPC_1P_v3_2014b/Rate Saturation Pitch2 ==
  data: u input; MinSaturation input; y_out output; MaxSaturation input; DT parameter
function y_out = fcn(u,MinSaturation,MaxSaturation,DT)
persistent y

if isempty(y)
    y = u;
end

rate = (u-y)/DT;
rate = min(max(rate,MinSaturation),MaxSaturation);

y = y + rate*DT;
y_out = y;
